simulink model "IEEE_39_IBR_Simplified"  (R2023b)
settings: Solver=FixedStepAuto  StartTime=0  StopTime=20  FixedStep=Ts  MaxStep=1/60  RelTol=1e-3  AbsTol=1e-2  EnableMultiTasking=on
PreLoadFcn:
  | NE39bus_data;
  | PSSMODEL=1;
  | LPSS=0;
  | WAPSS=0;
  | WAPSS2=0;
values from neighbouring files (symbols this model uses):
  Dt = 0    [SG_para.m]
  dw0_sm = 0    [SG_para.m]
  Emax = 1    [SG_para.m]
  Emin = 0.5    [SG_para.m]
  Fg = [0.1,0.1,0.1]    [SG_para.m]
  fn_sm = 60*ones(1,10)    [SG_para.m]
  H_sm = [5,3.03,3.58,2.86,2.6,3.48,2.64,2.43,3.45,4.2]*10    [SG_para.m]
  ia0_sm = 0.75*0    (= 0)    [SG_para.m]
  ib0_sm = 0.75*0    (= 0)    [SG_para.m]
  ic0_sm = 0.75*0    (= 0)    [SG_para.m]
  Kd_sm = 6*ones(1,10)    [SG_para.m]
  Ke = 200    [SG_para.m]
  Kg = [0.95,0.95,0.95]    [SG_para.m]
  Ks = 2    [SG_para.m]
  line = [     1	2	0.0035	0.0411	0.6987	0	100	345 ... (first row only)    [SG_para.m]
  p = 1    [SG_para.m]
  pha0_sm = -24.95*0    (= 0)    [SG_para.m]
  phb0_sm = -144.94*0    (= 0)    [SG_para.m]
  phc0_sm = 95.05*0    (= 0)    [SG_para.m]
  Pn_sm = [1000,1000,1000,1000,1000,1000,1000,1000,1000,1000]    [SG_para.m]
  Pref_sm = [1000 520.81 650 632 508 650 560 540 830 250]./Pn_sm    [SG_para.m]
  R = 1e-3    (= 0.001)    [SG_para.m]
  Rg = [0.05,0.05,0.05]    [SG_para.m]
  rs = 2.8544e-3    (= 0.0028544)    [SG_para.m]
  s = 1    [SG_para.m]
  s1 = 10    [SG_para.m]
  T1 = 0.05    [SG_para.m]
  T2 = 0.5    [SG_para.m]
  T3 = 0.5    [SG_para.m]
  Te = 0.05    [SG_para.m]
  Tfa = 3    [SG_para.m]
  Tfb = 10    [SG_para.m]
  Tg = [10,10,10]    [SG_para.m]
  theta0_sm = -94.3*0    (= 0)    [SG_para.m]
  Ts = 5e-5    (= 5e-05)    [SG_para.m]
  Ts1 = 0.18    [SG_para.m]
  Ts2 = 2    [SG_para.m]
  Ts3 = 5    [SG_para.m]
  Ts4 = 10    [SG_para.m]
  Ts5 = 15    [SG_para.m]
  Un_sm = [345,22,22,22,22,22,22,22,345,22]    [SG_para.m]
  Vmax = inf    [SG_para.m]
  Vmin = 0    [SG_para.m]
  Vref_sm = 1*ones(1,10)    [SG_para.m]
  xd = xd_t    (= 0.296)    [SG_para.m]
undefined symbols (not defined in the file or in its folder): D1, D11, Delta, Ka, Kf, Ta, Tf
libraries: spsThreePhaseVIMeasurementLib x41, spsThreePhaseFaultLib x39, spsThreePhaseSeriesRLCBranchLib x36, spsThreePhaseParallelRLCLoadLib x20, spsThreePhaseTransformerTwoWindingsLib x13, spsSimplifiedSynchronousMachinepuUnitsLib x10, spsLoadFlowBusLib x10, Inverter_based_Resources_IBRs x10, spsThreePhaseBreakerLib x2, spsSequenceAnalyzerLib x2, spsMultimeterLib x1, eePowerMeasurement x1
(part 2 of 5)

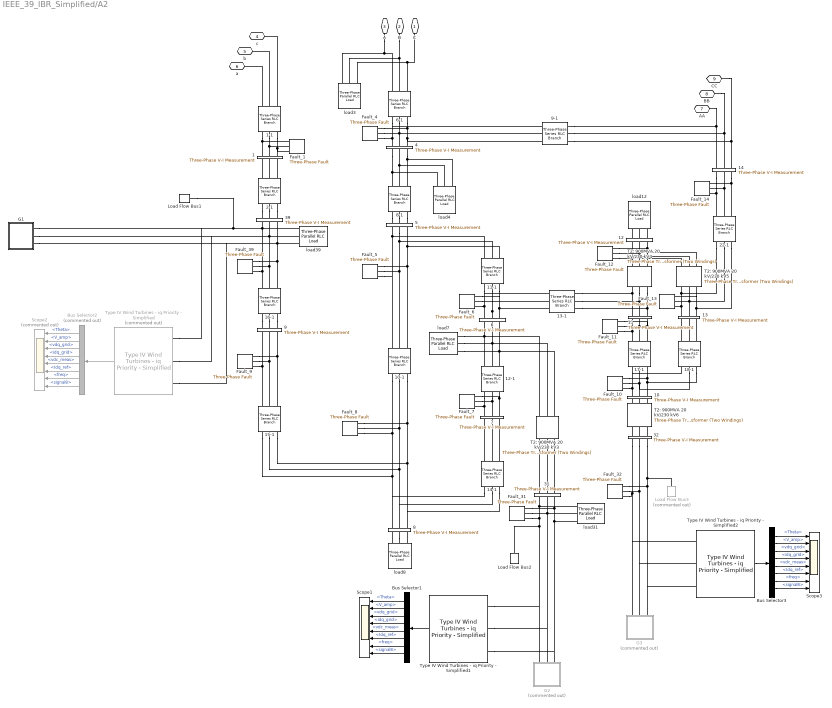
== system IEEE_39_IBR_Simplified/A2 ==
  1 : spsThreePhaseVIMeasurementLib/Three-Phase V-I Measurement  VoltageMeasurement=phase-to-phase  SetLabelV=on  LabelV=Vabc_1  Vpu=off  VpuLL=on  CurrentMeasurement=no  SetLabelI=on  LabelI=Iabc_B2  Ipu=off  Pbase=100e6  Vbase=Bus(1,2)*1e3  OutputType=Complex  PhasorSimulation=off  PSBequivalent=0
  1-1 : spsThreePhaseSeriesRLCBranchLib/Three-Phase Series RLC Branch  LConnTagsString=A|B|C  RConnTagsString=A|B|C  BranchType=RL  Resistance=line(1,3)  Inductance=line(1,4)  Capacitance=1e-6  Measurements=None
  10 : spsThreePhaseVIMeasurementLib/Three-Phase V-I Measurement  VoltageMeasurement=phase-to-phase  SetLabelV=on  LabelV=Vabc_10  Vpu=off  VpuLL=on  CurrentMeasurement=no  SetLabelI=on  LabelI=Iabc_B2  Ipu=off  Pbase=100e6  Vbase=Bus(10,2)*1e3  OutputType=Complex  PhasorSimulation=off  PSBequivalent=0
  10-1 : spsThreePhaseSeriesRLCBranchLib/Three-Phase Series RLC Branch  LConnTagsString=A|B|C  RConnTagsString=A|B|C  BranchType=RL  Resistance=line(10,3)  Inductance=line(10,4)  Capacitance=1e-6  Measurements=None
  11 : spsThreePhaseVIMeasurementLib/Three-Phase V-I Measurement  VoltageMeasurement=phase-to-phase  SetLabelV=on  LabelV=Vabc_11  Vpu=off  VpuLL=on  CurrentMeasurement=no  SetLabelI=on  LabelI=Iabc_B2  Ipu=off  Pbase=100e6  Vbase=Bus(11,2)*1e3  OutputType=Complex  PhasorSimulation=off  PSBequivalent=0
  11-1 : spsThreePhaseSeriesRLCBranchLib/Three-Phase Series RLC Branch  LConnTagsString=A|B|C  RConnTagsString=A|B|C  BranchType=RL  Resistance=line(11,3)  Inductance=line(11,4)  Capacitance=1e-6  Measurements=None
  12 : spsThreePhaseVIMeasurementLib/Three-Phase V-I Measurement  VoltageMeasurement=phase-to-phase  SetLabelV=on  LabelV=Vabc_12  Vpu=off  VpuLL=on  CurrentMeasurement=no  SetLabelI=on  LabelI=Iabc_B2  Ipu=off  Pbase=100e6  Vbase=Bus(12,2)*1e3  OutputType=Complex  PhasorSimulation=off  PSBequivalent=0
  12-1 : spsThreePhaseSeriesRLCBranchLib/Three-Phase Series RLC Branch  LConnTagsString=A|B|C  RConnTagsString=A|B|C  BranchType=RL  Resistance=line(12,3)  Inductance=line(12,4)  Capacitance=1e-6  Measurements=None
  13 : spsThreePhaseVIMeasurementLib/Three-Phase V-I Measurement  VoltageMeasurement=phase-to-phase  SetLabelV=on  LabelV=Vabc_13  Vpu=off  VpuLL=on  CurrentMeasurement=no  SetLabelI=on  LabelI=Iabc_B2  Ipu=off  Pbase=100e6  Vbase=Bus(13,2)*1e3  OutputType=Complex  PhasorSimulation=off  PSBequivalent=0
  13-1 : spsThreePhaseSeriesRLCBranchLib/Three-Phase Series RLC Branch  LConnTagsString=A|B|C  RConnTagsString=A|B|C  BranchType=RL  Resistance=line(13,3)  Inductance=line(13,4)  Capacitance=1e-6  Measurements=None
  14 : spsThreePhaseVIMeasurementLib/Three-Phase V-I Measurement  VoltageMeasurement=phase-to-phase  SetLabelV=on  LabelV=Vabc_14  Vpu=off  VpuLL=on  CurrentMeasurement=no  SetLabelI=on  LabelI=Iabc_B2  Ipu=off  Pbase=100e6  Vbase=Bus(14,2)*1e3  OutputType=Complex  PhasorSimulation=off  PSBequivalent=0
  14-1 : spsThreePhaseSeriesRLCBranchLib/Three-Phase Series RLC Branch  LConnTagsString=A|B|C  RConnTagsString=A|B|C  BranchType=RL  Resistance=line(14,3)  Inductance=line(14,4)  Capacitance=1e-6  Measurements=None
  15-1 : spsThreePhaseSeriesRLCBranchLib/Three-Phase Series RLC Branch  LConnTagsString=A|B|C  RConnTagsString=A|B|C  BranchType=RL  Resistance=line(15,3)  Inductance=line(15,4)  Capacitance=1e-6  Measurements=None
  16-1 : spsThreePhaseSeriesRLCBranchLib/Three-Phase Series RLC Branch  LConnTagsString=A|B|C  RConnTagsString=A|B|C  BranchType=RL  Resistance=line(16,3)  Inductance=line(16,4)  Capacitance=1e-6  Measurements=None
  17-1 : spsThreePhaseSeriesRLCBranchLib/Three-Phase Series RLC Branch  LConnTagsString=A|B|C  RConnTagsString=A|B|C  BranchType=RL  Resistance=line(17,3)  Inductance=line(17,4)  Capacitance=1e-6  Measurements=None
  18-1 : spsThreePhaseSeriesRLCBranchLib/Three-Phase Series RLC Branch  LConnTagsString=A|B|C  RConnTagsString=A|B|C  BranchType=RL  Resistance=line(18,3)  Inductance=line(18,4)  Capacitance=1e-6  Measurements=None
  2-1 : spsThreePhaseSeriesRLCBranchLib/Three-Phase Series RLC Branch  LConnTagsString=A|B|C  RConnTagsString=A|B|C  BranchType=RL  Resistance=line(2,3)  Inductance=line(2,4)  Capacitance=1e-6  Measurements=None
  22-1 : spsThreePhaseSeriesRLCBranchLib/Three-Phase Series RLC Branch  LConnTagsString=A|B|C  RConnTagsString=A|B|C  BranchType=RL  Resistance=line(22,3)  Inductance=line(22,4)  Capacitance=1e-6  Measurements=None
  31 : spsThreePhaseVIMeasurementLib/Three-Phase V-I Measurement  VoltageMeasurement=phase-to-phase  SetLabelV=on  LabelV=Vabc_31  Vpu=off  VpuLL=on  CurrentMeasurement=no  SetLabelI=on  LabelI=Iabc_B2  Ipu=off  Pbase=100e6  Vbase=Bus(31,2)*1e3  OutputType=Complex  PhasorSimulation=off  PSBequivalent=0
  32 : spsThreePhaseVIMeasurementLib/Three-Phase V-I Measurement  VoltageMeasurement=phase-to-phase  SetLabelV=on  LabelV=Vabc_32  Vpu=off  VpuLL=on  CurrentMeasurement=no  SetLabelI=on  LabelI=Iabc_B2  Ipu=off  Pbase=100e6  Vbase=Bus(32,2)*1e3  OutputType=Complex  PhasorSimulation=off  PSBequivalent=0
  39 : spsThreePhaseVIMeasurementLib/Three-Phase V-I Measurement  VoltageMeasurement=phase-to-phase  SetLabelV=on  LabelV=Vabc_39  Vpu=off  VpuLL=on  CurrentMeasurement=no  SetLabelI=on  LabelI=Iabc_B2  Ipu=off  Pbase=100e6  Vbase=Bus(39,2)*1e3  OutputType=Complex  PhasorSimulation=off  PSBequivalent=0
  4 : spsThreePhaseVIMeasurementLib/Three-Phase V-I Measurement  VoltageMeasurement=phase-to-phase  SetLabelV=on  LabelV=Vabc_B4  Vpu=off  VpuLL=on  CurrentMeasurement=yes  SetLabelI=on  LabelI=Iabc_B4  Ipu=off  Pbase=100e6  Vbase=Bus(4,2)*1e3  OutputType=Complex  PhasorSimulation=off  PSBequivalent=0
  5 : spsThreePhaseVIMeasurementLib/Three-Phase V-I Measurement  VoltageMeasurement=phase-to-phase  SetLabelV=on  LabelV=Vabc_5  Vpu=off  VpuLL=on  CurrentMeasurement=no  SetLabelI=on  LabelI=Iabc_B2  Ipu=off  Pbase=100e6  Vbase=Bus(5,2)*1e3  OutputType=Complex  PhasorSimulation=off  PSBequivalent=0
  6 : spsThreePhaseVIMeasurementLib/Three-Phase V-I Measurement  VoltageMeasurement=phase-to-phase  SetLabelV=on  LabelV=Vabc_6  Vpu=off  VpuLL=on  CurrentMeasurement=no  SetLabelI=on  LabelI=Iabc_B2  Ipu=off  Pbase=100e6  Vbase=Bus(6,2)*1e3  OutputType=Complex  PhasorSimulation=off  PSBequivalent=0
  6-1 : spsThreePhaseSeriesRLCBranchLib/Three-Phase Series RLC Branch  LConnTagsString=A|B|C  RConnTagsString=A|B|C  BranchType=RL  Resistance=line(6,3)  Inductance=line(6,4)  Capacitance=1e-6  Measurements=None
  7 : spsThreePhaseVIMeasurementLib/Three-Phase V-I Measurement  VoltageMeasurement=phase-to-phase  SetLabelV=on  LabelV=Vabc_7  Vpu=off  VpuLL=on  CurrentMeasurement=no  SetLabelI=on  LabelI=Iabc_B2  Ipu=off  Pbase=100e6  Vbase=Bus(8,2)*1e3  OutputType=Complex  PhasorSimulation=off  PSBequivalent=0
  8 : spsThreePhaseVIMeasurementLib/Three-Phase V-I Measurement  VoltageMeasurement=phase-to-phase  SetLabelV=on  LabelV=Vabc_8  Vpu=off  VpuLL=on  CurrentMeasurement=no  SetLabelI=on  LabelI=Iabc_B2  Ipu=off  Pbase=100e6  Vbase=Bus(8,2)*1e3  OutputType=Complex  PhasorSimulation=off  PSBequivalent=0
  8-1 : spsThreePhaseSeriesRLCBranchLib/Three-Phase Series RLC Branch  LConnTagsString=A|B|C  RConnTagsString=A|B|C  BranchType=RL  Resistance=line(8,3)  Inductance=line(8,4)  Capacitance=1e-6  Measurements=None
  9 : spsThreePhaseVIMeasurementLib/Three-Phase V-I Measurement  VoltageMeasurement=phase-to-phase  SetLabelV=on  LabelV=Vabc_9  Vpu=off  VpuLL=on  CurrentMeasurement=no  SetLabelI=on  LabelI=Iabc_B2  Ipu=off  Pbase=100e6  Vbase=Bus(9,2)*1e3  OutputType=Complex  PhasorSimulation=off  PSBequivalent=0
  9-1 : spsThreePhaseSeriesRLCBranchLib/Three-Phase Series RLC Branch  LConnTagsString=A|B|C  RConnTagsString=A|B|C  BranchType=RL  Resistance=line(9,3)  Inductance=line(9,4)  Capacitance=1e-6  Measurements=None
  Bus Selector1 : BusSelector  OutputSignals=Theta,V_amp,vdq_grid,idq_grid,vdc_meas,Idq_ref,freq,signal8
  Bus Selector2 : BusSelector  Commented=on  OutputSignals=Theta,V_amp,vdq_grid,idq_grid,vdc_meas,Idq_ref,freq,signal8
  Bus Selector3 : BusSelector  OutputSignals=Theta,V_amp,vdq_grid,idq_grid,vdc_meas,Idq_ref,freq,signal8
  Fault_1 : spsThreePhaseFaultLib/Three-Phase Fault  InitialStates=0  FaultA=on  FaultB=on  FaultC=on  GroundFault=on  SwitchTimes="[t(1)+1/60  t(1)+5/60]"  External=off  SwitchStatus=NaN  FaultResistance=0.001  GroundResistance=0.01  SnubberResistance=1e6  SnubberCapacitance=inf  Measurements=Fault voltages and currents
  Fault_10 : spsThreePhaseFaultLib/Three-Phase Fault  InitialStates=0  FaultA=on  FaultB=on  FaultC=on  GroundFault=on  SwitchTimes="[t(10)+1/60  t(10)+5/60]"  External=off  SwitchStatus=NaN  FaultResistance=0.001  GroundResistance=0.01  SnubberResistance=1e6  SnubberCapacitance=inf  Measurements=Fault voltages and currents
  Fault_11 : spsThreePhaseFaultLib/Three-Phase Fault  InitialStates=0  FaultA=on  FaultB=on  FaultC=on  GroundFault=on  SwitchTimes="[t(11)+1/60  t(11)+5/60]"  External=off  SwitchStatus=NaN  FaultResistance=0.001  GroundResistance=0.01  SnubberResistance=1e6  SnubberCapacitance=inf  Measurements=Fault voltages and currents
  Fault_12 : spsThreePhaseFaultLib/Three-Phase Fault  InitialStates=0  FaultA=on  FaultB=on  FaultC=on  GroundFault=on  SwitchTimes="[t(12)+1/60  t(12)+5/60]"  External=off  SwitchStatus=NaN  FaultResistance=0.001  GroundResistance=0.01  SnubberResistance=1e6  SnubberCapacitance=inf  Measurements=Fault voltages and currents
  Fault_13 : spsThreePhaseFaultLib/Three-Phase Fault  InitialStates=0  FaultA=on  FaultB=on  FaultC=on  GroundFault=on  SwitchTimes="[t(13)+1/60  t(13)+5/60]"  External=off  SwitchStatus=NaN  FaultResistance=0.001  GroundResistance=0.01  SnubberResistance=1e6  SnubberCapacitance=inf  Measurements=Fault voltages and currents
  Fault_14 : spsThreePhaseFaultLib/Three-Phase Fault  InitialStates=0  FaultA=on  FaultB=on  FaultC=on  GroundFault=on  SwitchTimes="[t(14)+1/60  t(14)+5/60]"  External=off  SwitchStatus=NaN  FaultResistance=0.001  GroundResistance=0.01  SnubberResistance=1e6  SnubberCapacitance=inf  Measurements=Fault voltages and currents
  Fault_31 : spsThreePhaseFaultLib/Three-Phase Fault  InitialStates=0  FaultA=on  FaultB=on  FaultC=on  GroundFault=on  SwitchTimes="[t(31)+1/60  t(31)+5/60]"  External=off  SwitchStatus=NaN  FaultResistance=0.001  GroundResistance=0.01  SnubberResistance=1e6  SnubberCapacitance=inf  Measurements=Fault voltages and currents
  Fault_32 : spsThreePhaseFaultLib/Three-Phase Fault  InitialStates=0  FaultA=on  FaultB=on  FaultC=on  GroundFault=on  SwitchTimes="[t(32)+1/60  t(32)+5/60]"  External=off  SwitchStatus=NaN  FaultResistance=0.001  GroundResistance=0.01  SnubberResistance=1e6  SnubberCapacitance=inf  Measurements=Fault voltages and currents
  Fault_39 : spsThreePhaseFaultLib/Three-Phase Fault  InitialStates=0  FaultA=on  FaultB=on  FaultC=on  GroundFault=on  SwitchTimes="[t(39)+1/60  t(39)+5/60]"  External=off  SwitchStatus=NaN  FaultResistance=0.001  GroundResistance=0.01  SnubberResistance=1e6  SnubberCapacitance=inf  Measurements=Fault voltages and currents
  Fault_4 : spsThreePhaseFaultLib/Three-Phase Fault  InitialStates=0  FaultA=on  FaultB=on  FaultC=on  GroundFault=on  SwitchTimes="[t(4)+1/60  t(4)+5/60]"  External=off  SwitchStatus=NaN  FaultResistance=0.001  GroundResistance=0.01  SnubberResistance=1e6  SnubberCapacitance=inf  Measurements=Fault voltages and currents
  Fault_5 : spsThreePhaseFaultLib/Three-Phase Fault  InitialStates=0  FaultA=on  FaultB=on  FaultC=on  GroundFault=on  SwitchTimes="[t(5)+1/60  t(5)+5/60]"  External=off  SwitchStatus=NaN  FaultResistance=0.001  GroundResistance=0.01  SnubberResistance=1e6  SnubberCapacitance=inf  Measurements=Fault voltages and currents
  Fault_6 : spsThreePhaseFaultLib/Three-Phase Fault  InitialStates=0  FaultA=on  FaultB=on  FaultC=on  GroundFault=on  SwitchTimes="[t(6)+1/60  t(6)+5/60]"  External=off  SwitchStatus=NaN  FaultResistance=0.001  GroundResistance=0.01  SnubberResistance=1e6  SnubberCapacitance=inf  Measurements=Fault voltages and currents
  Fault_7 : spsThreePhaseFaultLib/Three-Phase Fault  InitialStates=0  FaultA=on  FaultB=on  FaultC=on  GroundFault=on  SwitchTimes="[t(7)+1/60  t(7)+5/60]"  External=off  SwitchStatus=NaN  FaultResistance=0.001  GroundResistance=0.01  SnubberResistance=1e6  SnubberCapacitance=inf  Measurements=Fault voltages and currents
  Fault_8 : spsThreePhaseFaultLib/Three-Phase Fault  InitialStates=0  FaultA=on  FaultB=on  FaultC=on  GroundFault=on  SwitchTimes="[t(8)+1/60  t(8)+5/60]"  External=off  SwitchStatus=NaN  FaultResistance=0.001  GroundResistance=0.01  SnubberResistance=1e6  SnubberCapacitance=inf  Measurements=Fault voltages and currents
  Fault_9 : spsThreePhaseFaultLib/Three-Phase Fault  InitialStates=0  FaultA=on  FaultB=on  FaultC=on  GroundFault=on  SwitchTimes="[t(9)+1/60  t(9)+5/60]"  External=off  SwitchStatus=NaN  FaultResistance=0.001  GroundResistance=0.01  SnubberResistance=1e6  SnubberCapacitance=inf  Measurements=Fault voltages and currents
  G1 : Subsystem
  G2 : Subsystem  Commented=on
  G3 : Subsystem  Commented=on
  Load Flow Bus1 : spsLoadFlowBusLib/Load Flow Bus  LConnTagsString=a  Phases=single  Connectors=on one side  ID=Bus39  Vbase=345e3  Vref=1.03  Vangle=0  VLF=1.03  VLFb=1  VLFc=1  angleLF=19.62  angleLFb=0  angleLFc=0
      settings: AttributesFormatString=%<ID>\n%<Vbase>V\n%<VLF>pu\n%<angleLF>deg.
  Load Flow Bus2 : spsLoadFlowBusLib/Load Flow Bus  LConnTagsString=a  Phases=single  Connectors=on one side  ID=Bus31  Vbase=22e3  Vref=0.9820  Vangle=0  VLF=0.982  VLFb=1  VLFc=1  angleLF=0  angleLFb=0  angleLFc=0
      settings: AttributesFormatString=%<ID>\n%<Vbase>V\n%<VLF>pu\n%<angleLF>deg.
  Load Flow Bus3 : spsLoadFlowBusLib/Load Flow Bus  Commented=on  LConnTagsString=a  Phases=single  Connectors=on one side  ID=Bus32  Vbase=22e3  Vref=0.9831  Vangle=0  VLF=0.9831  VLFb=1  VLFc=1  angleLF=2.466  angleLFb=0  angleLFc=0
      settings: AttributesFormatString=%<ID>\n%<Vbase>V\n%<VLF>pu\n%<angleLF>deg.
  Scope1 : Scope  NumInputPorts=8
  Scope2 : Scope  Commented=on  NumInputPorts=8
  Scope3 : Scope  NumInputPorts=8
  T2: 900MVA 20 kV/230 kV3 : spsThreePhaseTransformerTwoWindingsLib/Three-Phase Transformer (Two Windings)  Winding1Connection=Delta (D1)  Winding2Connection=Yg  CoreType=Three single-phase transformers  SetSaturation=off  Hysteresis=off  DataFile='hysteresis'  SetInitialFlux=off  Measurements=None  UNITS=pu  NominalPower=[ 1000e6 60 ]  Winding1="[ 22e3*1.0 1e-6  0]"  Winding2="[ 345e3*1.0  1e-6  0.0250*s ]"  Rm=500  Lm=500  L0=0.5  Saturation="[ 0,0  ;  0.005,1.2  ;  1.0,1.4 ]"  InitialFluxes=[ 0.8 , -0.8 , 0.7 ]  BreakLoop=off  DiscreteSolver=Trapezoidal iterative  DataType=off  TransfoNumber=0
  T2: 900MVA 20 kV/230 kV4 : spsThreePhaseTransformerTwoWindingsLib/Three-Phase Transformer (Two Windings)  Winding1Connection=Y  Winding2Connection=Y  CoreType=Three single-phase transformers  SetSaturation=off  Hysteresis=off  DataFile='hysteresis'  SetInitialFlux=off  Measurements=None  UNITS=pu  NominalPower=[ 1000e6 60 ]  Winding1="[ 345e3 .0008*s  0]"  Winding2="[ 230e3*1.00  .0008*s   .0435*s1]"  Rm=500  Lm=500  L0=0.5  Saturation="[ 0,0  ;  0.005,1.2  ;  1.0,1.4 ]"  InitialFluxes=[ 0.8 , -0.8 , 0.7 ]  BreakLoop=off  DiscreteSolver=Trapezoidal iterative  DataType=off  TransfoNumber=0
  T2: 900MVA 20 kV/230 kV5 : spsThreePhaseTransformerTwoWindingsLib/Three-Phase Transformer (Two Windings)  Winding1Connection=Y  Winding2Connection=Y  CoreType=Three single-phase transformers  SetSaturation=off  Hysteresis=off  DataFile='hysteresis'  SetInitialFlux=off  Measurements=None  UNITS=pu  NominalPower=[ 1000e6 60 ]  Winding1="[ 345e3 .0008*s  0]"  Winding2="[ 230e3*1.00 .0008*s  .0435*s1]"  Rm=500  Lm=500  L0=0.5  Saturation="[ 0,0  ;  0.005,1.2  ;  1.0,1.4 ]"  InitialFluxes=[ 0.8 , -0.8 , 0.7 ]  BreakLoop=off  DiscreteSolver=Trapezoidal iterative  DataType=off  TransfoNumber=0
  T2: 900MVA 20 kV/230 kV6 : spsThreePhaseTransformerTwoWindingsLib/Three-Phase Transformer (Two Windings)  Winding1Connection=Delta (D1)  Winding2Connection=Yg  CoreType=Three single-phase transformers  SetSaturation=off  Hysteresis=off  DataFile='hysteresis'  SetInitialFlux=off  Measurements=None  UNITS=pu  NominalPower=[ 1000e6 60 ]  Winding1="[ 22e3*1.0 1e-6  0]"  Winding2="[ 345e3*1.0   1e-6    0.020*s ]"  Rm=500  Lm=500  L0=0.5  Saturation="[ 0,0  ;  0.005,1.2  ;  1.0,1.4 ]"  InitialFluxes=[ 0.8 , -0.8 , 0.7 ]  BreakLoop=off  DiscreteSolver=Trapezoidal iterative  DataType=off  TransfoNumber=0
  Type IV Wind Turbines - iq Priority - Simplified : Inverter_based_Resources_IBRs/Inverter-based Resources (IBRs)/Type IV Wind Turbines - iq Priority - Simplified  Commented=on  Num_WTs=1  Wind_Speed_WT=15  Q_ref_pu_WT=0  Transformer_P_f="[1000e6  60]"  Transformer_V1_R1_L1=[345e3*1.05 , 0.025/30 , 0.025]  DC_Power=1000e6*0.97
  Type IV Wind Turbines - iq Priority - Simplified1 : Inverter_based_Resources_IBRs/Inverter-based Resources (IBRs)/Type IV Wind Turbines - iq Priority - Simplified  Num_WTs=1  Wind_Speed_WT=15  Q_ref_pu_WT=0  Transformer_P_f="[1000e6  60]"  Transformer_V1_R1_L1=[22e3 , 0.025/30 , 0.025]  DC_Power=1000e6*0.381
  Type IV Wind Turbines - iq Priority - Simplified2 : Inverter_based_Resources_IBRs/Inverter-based Resources (IBRs)/Type IV Wind Turbines - iq Priority - Simplified  Num_WTs=1  Wind_Speed_WT=15  Q_ref_pu_WT=0  Transformer_P_f="[1000e6  60]"  Transformer_V1_R1_L1=[22e3 , 0.025/30 , 0.025]  DC_Power=1000e6*0.5092
  load12 : spsThreePhaseParallelRLCLoadLib/Three-Phase Parallel RLC Load  LConnTagsString=A|B|C  Configuration=Y (grounded)  NominalVoltage=(230000)*0.939625  Vabc=[1e3 1e3 1e3]  Vabcp=[1e3 1e3 1e3]  NominalFrequency=60  UnbalancedPower=off  ActivePower=7.5e6  InductivePower=88e6  CapacitivePower=0  Pabc=[10e3 9e3 11e3]  QLabc=[100 90 110]  QCabc=[100 90 110]  Pabcp=[10e3 9e3 11e3]  QLabcp=[100 90 110]  QCabcp=[100 90 110]  Measurements=None  LoadType=constant PQ
  load3 : spsThreePhaseParallelRLCLoadLib/Three-Phase Parallel RLC Load  LConnTagsString=A|B|C  Configuration=Y (grounded)  NominalVoltage=(345000)*0.992094  Vabc=[1e3 1e3 1e3]  Vabcp=[1e3 1e3 1e3]  NominalFrequency=60  UnbalancedPower=off  ActivePower=322e6  InductivePower=2.4e6  CapacitivePower=0  Pabc=[10e3 9e3 11e3]  QLabc=[100 90 110]  QCabc=[100 90 110]  Pabcp=[10e3 9e3 11e3]  QLabcp=[100 90 110]  QCabcp=[100 90 110]  Measurements=None  LoadType=constant PQ
  load31 : spsThreePhaseParallelRLCLoadLib/Three-Phase Parallel RLC Load  LConnTagsString=A|B|C  Configuration=Y (grounded)  NominalVoltage=(22000)*0.982  Vabc=[1e3 1e3 1e3]  Vabcp=[1e3 1e3 1e3]  NominalFrequency=60  UnbalancedPower=off  ActivePower=9.2e6  InductivePower=4.6e6  CapacitivePower=0  Pabc=[10e3 9e3 11e3]  QLabc=[100 90 110]  QCabc=[100 90 110]  Pabcp=[10e3 9e3 11e3]  QLabcp=[100 90 110]  QCabcp=[100 90 110]  Measurements=None  LoadType=constant PQ
  load39 : spsThreePhaseParallelRLCLoadLib/Three-Phase Parallel RLC Load  LConnTagsString=A|B|C  Configuration=Y (grounded)  NominalVoltage=(345000)*1.03  Vabc=[1e3 1e3 1e3]  Vabcp=[1e3 1e3 1e3]  NominalFrequency=60  UnbalancedPower=off  ActivePower=1104e6  InductivePower=250e6  CapacitivePower=0  Pabc=[10e3 9e3 11e3]  QLabc=[100 90 110]  QCabc=[100 90 110]  Pabcp=[10e3 9e3 11e3]  QLabcp=[100 90 110]  QCabcp=[100 90 110]  Measurements=None  LoadType=constant PQ
  load4 : spsThreePhaseParallelRLCLoadLib/Three-Phase Parallel RLC Load  LConnTagsString=A|B|C  Configuration=Y (grounded)  NominalVoltage=(345000)*0.95637  Vabc=[1e3 1e3 1e3]  Vabcp=[1e3 1e3 1e3]  NominalFrequency=60  UnbalancedPower=off  ActivePower=500e6  InductivePower=184e6  CapacitivePower=0  Pabc=[10e3 9e3 11e3]  QLabc=[100 90 110]  QCabc=[100 90 110]  Pabcp=[10e3 9e3 11e3]  QLabcp=[100 90 110]  QCabcp=[100 90 110]  Measurements=None  LoadType=constant PQ
  load7 : spsThreePhaseParallelRLCLoadLib/Three-Phase Parallel RLC Load  LConnTagsString=A|B|C  Configuration=Y (grounded)  NominalVoltage=(345000)*0.956463  Vabc=[1e3 1e3 1e3]  Vabcp=[1e3 1e3 1e3]  NominalFrequency=60  UnbalancedPower=off  ActivePower=233e6  InductivePower=84e6  CapacitivePower=0  Pabc=[10e3 9e3 11e3]  QLabc=[100 90 110]  QCabc=[100 90 110]  Pabcp=[10e3 9e3 11e3]  QLabcp=[100 90 110]  QCabcp=[100 90 110]  Measurements=None  LoadType=constant PQ
  load8 : spsThreePhaseParallelRLCLoadLib/Three-Phase Parallel RLC Load  LConnTagsString=A|B|C  Configuration=Y (grounded)  NominalVoltage=(345000)*0.954036  Vabc=[1e3 1e3 1e3]  Vabcp=[1e3 1e3 1e3]  NominalFrequency=60  UnbalancedPower=off  ActivePower=522e6  InductivePower=176e6  CapacitivePower=0  Pabc=[10e3 9e3 11e3]  QLabc=[100 90 110]  QCabc=[100 90 110]  Pabcp=[10e3 9e3 11e3]  QLabcp=[100 90 110]  QCabcp=[100 90 110]  Measurements=None  LoadType=constant PQ
  C : PMIOPort  Side=Left
  B : PMIOPort  Port=2  Side=Left
  A : PMIOPort  Port=3  Side=Left
  c : PMIOPort  Port=4  Side=Left
  b : PMIOPort  Port=5  Side=Left
  a : PMIOPort  Port=6  Side=Left
  AA : PMIOPort  Port=7  Side=Right
  BB : PMIOPort  Port=8  Side=Right
  CC : PMIOPort  Port=9  Side=Right
  wires:
  Bus Selector2/3 -> Scope2/3  "<vdq_grid>"
  Bus Selector2/2 -> Scope2/2  "<V_amp>"
  Bus Selector2/4 -> Scope2/4  "<idq_grid>"
  Bus Selector2/5 -> Scope2/5  "<vdc_meas>"
  Bus Selector2/6 -> Scope2/6  "<Idq_ref>"
  Bus Selector2/1 -> Scope2/1  "<Theta>"
  Bus Selector2/8 -> Scope2/8  "<signal8>"
  Type IV Wind Turbines - iq Priority - Simplified/1 -> Bus Selector2/1
  Bus Selector2/7 -> Scope2/7  "<freq>"
  Bus Selector1/3 -> Scope1/3  "<vdq_grid>"
  Bus Selector1/2 -> Scope1/2  "<V_amp>"
  Bus Selector1/4 -> Scope1/4  "<idq_grid>"
  Bus Selector1/5 -> Scope1/5  "<vdc_meas>"
  Bus Selector1/6 -> Scope1/6  "<Idq_ref>"
  Bus Selector1/1 -> Scope1/1  "<Theta>"
  Bus Selector1/8 -> Scope1/8  "<signal8>"
  Type IV Wind Turbines - iq Priority - Simplified1/1 -> Bus Selector1/1
  Bus Selector1/7 -> Scope1/7  "<freq>"
  Bus Selector3/5 -> Scope3/5  "<vdc_meas>"
  Bus Selector3/4 -> Scope3/4  "<idq_grid>"
  Bus Selector3/7 -> Scope3/7  "<freq>"
  Bus Selector3/8 -> Scope3/8  "<signal8>"
  Type IV Wind Turbines - iq Priority - Simplified2/1 -> Bus Selector3/1
  Bus Selector3/1 -> Scope3/1  "<Theta>"
  Bus Selector3/6 -> Scope3/6  "<Idq_ref>"
  Bus Selector3/3 -> Scope3/3  "<vdq_grid>"
  Bus Selector3/2 -> Scope3/2  "<V_amp>"
  connections:
  load3/LConn3 -- 6-1/LConn3 -- C/RConn1
  Fault_11/LConn1 -- 17-1/LConn1 -- 11/RConn1
  5/RConn2 -- 11-1/LConn2 -- 10-1/LConn2 -- Fault_5/LConn2
  14-1/LConn1 -- 7/LConn1
  Fault_8/LConn3 -- 14-1/RConn3 -- 8/LConn3 -- 15-1/RConn3 -- 10-1/RConn3
  load8/LConn1 -- 8/RConn1
  14-1/LConn2 -- 7/LConn2
  18-1/LConn2 -- 13/RConn2
  2-1/LConn2 -- 1/RConn2
  Fault_8/LConn2 -- 14-1/RConn2 -- 8/LConn2 -- 15-1/RConn2 -- 10-1/RConn2
  T2: 900MVA 20 kV/230 kV6/RConn1 -- 10/RConn1
  9-1/LConn3 -- CC/RConn1 -- 14/RConn3
  Fault_1/LConn1 -- 1-1/RConn1 -- 1/LConn1
  T2: 900MVA 20 kV/230 kV3/RConn1 -- 12-1/LConn1 -- load7/LConn1 -- 6/RConn1
  2-1/LConn3 -- 1/RConn3
  T2: 900MVA 20 kV/230 kV4/RConn1 -- Fault_12/LConn1 -- T2: 900MVA 20 kV/230 kV5/RConn1 -- 12/RConn1
  Fault_7/LConn1 -- 12-1/RConn1 -- 7/RConn1
  39/RConn1 -- load39/LConn1 -- Type IV Wind Turbines - iq Priority - Simplified/LConn1 -- G1/LConn1 -- Load Flow Bus1/LConn1 -- 16-1/LConn1 -- Fault_39/LConn1
  load31/LConn3 -- Type IV Wind Turbines - iq Priority - Simplified1/LConn3 -- G2/LConn3 -- Fault_31/LConn3 -- 31/RConn3
  T2: 900MVA 20 kV/230 kV4/LConn2 -- 13-1/RConn2 -- 11/LConn2
  Fault_8/LConn1 -- 8/LConn1 -- 14-1/RConn1 -- 15-1/RConn1 -- 10-1/RConn1
  Fault_9/LConn3 -- 15-1/LConn3 -- 9/RConn3
  Fault_1/LConn3 -- 1-1/RConn3 -- 1/LConn3
  T2: 900MVA 20 kV/230 kV4/RConn3 -- T2: 900MVA 20 kV/230 kV5/RConn3 -- Fault_12/LConn3 -- 12/RConn3
  13-1/LConn1 -- 11-1/RConn1 -- 6/LConn1 -- Fault_6/LConn1
  32/RConn1 -- Type IV Wind Turbines - iq Priority - Simplified2/LConn1 -- G3/LConn1 -- Fault_32/LConn1
  32/RConn3 -- Load Flow Bus3/LConn1 -- Type IV Wind Turbines - iq Priority - Simplified2/LConn3 -- G3/LConn3 -- Fault_32/LConn3
  Fault_10/LConn3 -- 17-1/RConn3 -- 18-1/RConn3 -- 10/LConn3
  6/RConn3 -- 12-1/LConn3 -- T2: 900MVA 20 kV/230 kV3/RConn3 -- load7/LConn3
  6/LConn2 -- 13-1/LConn2 -- 11-1/RConn2 -- Fault_6/LConn2
  9-1/LConn1 -- AA/RConn1 -- 14/RConn1
  Fault_11/LConn3 -- 17-1/LConn3 -- 11/RConn3
  load3/LConn2 -- B/RConn1 -- 6-1/LConn2
  2-1/RConn2 -- 39/LConn2
  13/LConn1 -- Fault_13/LConn1 -- 22-1/RConn1 -- T2: 900MVA 20 kV/230 kV5/LConn1
  14/LConn3 -- 22-1/LConn3 -- Fault_14/LConn3
  18-1/LConn1 -- 13/RConn1
  Fault_13/LConn3 -- T2: 900MVA 20 kV/230 kV5/LConn3 -- 22-1/RConn3 -- 13/LConn3
  18-1/LConn3 -- 13/RConn3
  Fault_39/LConn2 -- 16-1/LConn2 -- Type IV Wind Turbines - iq Priority - Simplified/LConn2 -- G1/LConn2 -- load39/LConn2 -- 39/RConn2
  13/LConn2 -- 22-1/RConn2 -- Fault_13/LConn2 -- T2: 900MVA 20 kV/230 kV5/LConn2
  2-1/RConn1 -- 39/LConn1
  Fault_14/LConn2 -- 22-1/LConn2 -- 14/LConn2
  Fault_4/LConn2 -- 9-1/RConn2 -- 6-1/RConn2 -- 4/LConn2
  Fault_11/LConn2 -- 17-1/LConn2 -- 11/RConn2
  17-1/RConn1 -- 18-1/RConn1 -- Fault_10/LConn1 -- 10/LConn1
  Fault_9/LConn2 -- 15-1/LConn2 -- 9/RConn2
  Fault_9/LConn1 -- 15-1/LConn1 -- 9/RConn1
  14/LConn1 -- 22-1/LConn1 -- Fault_14/LConn1
  load3/LConn1 -- 6-1/LConn1 -- A/RConn1
  Fault_4/LConn3 -- 6-1/RConn3 -- 9-1/RConn3 -- 4/LConn3
  1-1/LConn2 -- b/RConn1
  9-1/RConn1 -- 6-1/RConn1 -- Fault_4/LConn1 -- 4/LConn1
  Fault_10/LConn2 -- 17-1/RConn2 -- 18-1/RConn2 -- 10/LConn2
  31/LConn2 -- T2: 900MVA 20 kV/230 kV3/LConn2
  2-1/RConn3 -- 39/LConn3
  32/LConn1 -- T2: 900MVA 20 kV/230 kV6/LConn1
  9-1/LConn2 -- BB/RConn1 -- 14/RConn2
  Fault_1/LConn2 -- 1-1/RConn2 -- 1/LConn2
  10-1/LConn1 -- Fault_5/LConn1 -- 11-1/LConn1 -- 5/RConn1
  2-1/LConn1 -- 1/RConn1
  16-1/RConn1 -- 9/LConn1
  14-1/LConn3 -- 7/LConn3
  4/RConn1 -- 8-1/LConn1 -- load4/LConn1
  Fault_5/LConn3 -- 10-1/LConn3 -- 11-1/LConn3 -- 5/RConn3
  Fault_39/LConn3 -- 16-1/LConn3 -- Type IV Wind Turbines - iq Priority - Simplified/LConn3 -- G1/LConn3 -- load39/LConn3 -- 39/RConn3
  T2: 900MVA 20 kV/230 kV3/RConn2 -- 12-1/LConn2 -- load7/LConn2 -- 6/RConn2
  load31/LConn2 -- Type IV Wind Turbines - iq Priority - Simplified1/LConn2 -- G2/LConn2 -- Fault_31/LConn2 -- 31/RConn2
  32/LConn2 -- T2: 900MVA 20 kV/230 kV6/LConn2
  Fault_7/LConn2 -- 12-1/RConn2 -- 7/RConn2
  8-1/RConn1 -- 5/LConn1
  load4/LConn2 -- 8-1/LConn2 -- 4/RConn2
  16-1/RConn3 -- 9/LConn3
  16-1/RConn2 -- 9/LConn2
  Load Flow Bus2/LConn1 -- Type IV Wind Turbines - iq Priority - Simplified1/LConn1 -- G2/LConn1 -- Fault_31/LConn1 -- load31/LConn1 -- 31/RConn1
  4/RConn3 -- 8-1/LConn3 -- load4/LConn3
  8-1/RConn3 -- 5/LConn3
  32/RConn2 -- Type IV Wind Turbines - iq Priority - Simplified2/LConn2 -- G3/LConn2 -- Fault_32/LConn2
  8-1/RConn2 -- 5/LConn2
  11-1/RConn3 -- Fault_6/LConn3 -- 13-1/LConn3 -- 6/LConn3
  T2: 900MVA 20 kV/230 kV4/LConn3 -- 13-1/RConn3 -- 11/LConn3
  12/LConn2 -- load12/LConn2
  12/LConn3 -- load12/LConn3
  31/LConn1 -- T2: 900MVA 20 kV/230 kV3/LConn1
  8/RConn2 -- load8/LConn2
  load8/LConn3 -- 8/RConn3
  32/LConn3 -- T2: 900MVA 20 kV/230 kV6/LConn3
  Fault_7/LConn3 -- 12-1/RConn3 -- 7/RConn3
  T2: 900MVA 20 kV/230 kV4/RConn2 -- T2: 900MVA 20 kV/230 kV5/RConn2 -- Fault_12/LConn2 -- 12/RConn2
  31/LConn3 -- T2: 900MVA 20 kV/230 kV3/LConn3
  T2: 900MVA 20 kV/230 kV6/RConn3 -- 10/RConn3
  10/RConn2 -- T2: 900MVA 20 kV/230 kV6/RConn2
  T2: 900MVA 20 kV/230 kV4/LConn1 -- 13-1/RConn1 -- 11/LConn1
  12/LConn1 -- load12/LConn1
  1-1/LConn3 -- c/RConn1
  1-1/LConn1 -- a/RConn1
